simulink model "zzw_pcopy_offline2018"  (R2018b)
settings: Solver=VariableStepAuto  StartTime=0.0  StopTime=200  RelTol=1e-3
settings Model: Creator=Administrator  LastModifiedBy=anc
settings OptimizationCC: LifeSpan=inf
settings SFSimCC: SimUseLocalCustomCode=off
settings RTWCC: RTWUseLocalCustomCode=off
settings CodeAppCC: StateflowObjectComments=on

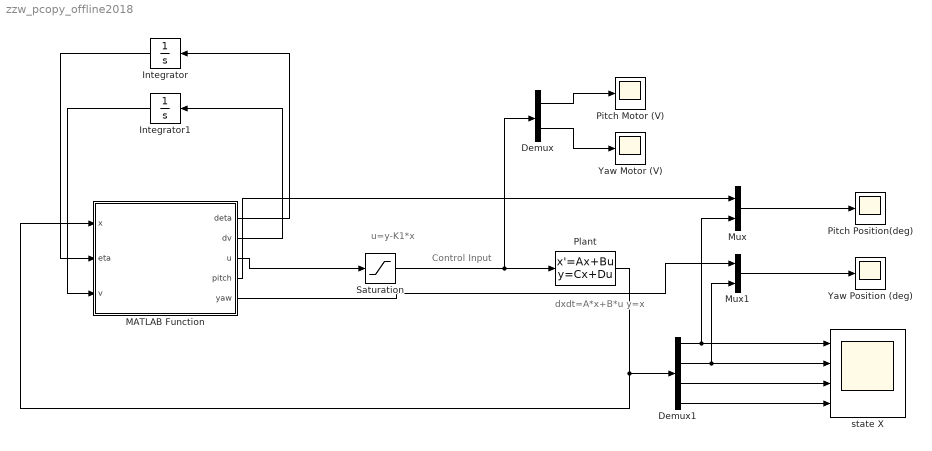
== system zzw_pcopy_offline2018 ==
  note: Control Input
  note: dxdt=A*x+B*u
      |      y=x
  note: u=y-K1*x
  Demux : Demux  Outputs=2
  Demux1 : Demux
  Integrator : Integrator  InitialCondition=[0;0;0;0]
  Integrator1 : Integrator  InitialCondition=[0;0.5*0.1*pi;0.5;0]
  MATLAB Function : MATLAB Function  TreatAsAtomicUnit=on
  Mux : Mux  Inputs=2
  Mux1 : Mux  Inputs=2
  Pitch Motor (V) : Scope
  Pitch Position(deg) : Scope
  Plant : StateSpace  A=[0 0 1 0;0 0 0 1;-1.7117 0 -0.3249 0;0 0 0 -1.0004]  B=[0 0;0 0;0.0503 0.0959;-0.1228 0.1]  C=[1 0 0 0;0 1 0 0;0 0 1 0;0 0 0 1]  D=[0 0;0 0;0 0;0 0]  InitialCondition=[2 1 0 0]
  Saturation : Saturate  UpperLimit=24  LowerLimit=-24
  Yaw Motor (V) : Scope
  Yaw Position (deg) : Scope
  state X : Scope  NumInputPorts=4
  wires:
  Demux1/3 -> state X/3
  Plant/1 -> Demux1/1, MATLAB Function/1(x)
  Demux1/1 -> state X/1, Mux/2
  Demux/2 -> Yaw Motor (V)/1
  Mux/1 -> Pitch Position(deg)/1
  Demux1/4 -> state X/4
  MATLAB Function/3(u) -> Saturation/1
  Mux1/1 -> Yaw Position (deg)/1
  Demux/1 -> Pitch Motor (V)/1
  Demux1/2 -> state X/2, Mux1/2
  MATLAB Function/1(deta) -> Integrator/1
  MATLAB Function/2(dv) -> Integrator1/1
  Integrator/1 -> MATLAB Function/2(eta)
  Integrator1/1 -> MATLAB Function/3(v)
  MATLAB Function/4(pitch) -> Mux/1
  MATLAB Function/5(yaw) -> Mux1/1
  Saturation/1 -> Plant/1, Demux/1

== matlab function zzw_pcopy_offline2018/MATLAB Function ==
  data: deta output; x input; eta input; dv output; v input; u output; pitch output; yaw output
function [deta,dv,u,pitch,yaw] = fcn(x,eta,v)

k1=5;
k2=2;

omega = 0.1*pi;
S=[0 1 0 0;
    -omega^2 0 0 0;
    0 0 0 1;
    0 0 -omega^2 0];
ex=zeros(2,1);
ev=zeros(2,1);

ex(1)=x(1)-v(1);
ex(2)=x(2)-v(3);

ev(1)=x(3)-v(2);
ev(2)=x(4)-v(4);


M=[0 1;
    -0.7017 -0.7017];
N=[0;1];
phi=[0 1;-omega^2 0];

psi=[1 0];

a=-M;
b=phi;
c=N*psi;
%T=sylvester(a,b,c);
T=[1.4629 -1.7023;
   0.1680 1.4629];
ep=k2*ex+ev;

us=zeros(2,1);                                                                                                                   
us(1)= -k1*(1+ep(1)^2)*ep(1)+psi*inv(T)*eta(1:2);
us(2)= -k1*(1+ep(2)^2)*ep(2)+psi*inv(T)*eta(3:4);

R=[0.0503 0.0959;
    -0.1228 0.1];
u=zeros(2,1);
u=inv(R)*us;

pitch=x(1);
yaw=x(2);

dv=zeros(4,1);
deta = zeros(4,1);
dv=S*v;
deta(1:2)=M*eta(1:2)+N*us(1);
deta(3:4)=M*eta(3:4)+N*us(2);
end
